simulink model "projeto_final_simulink"  (R2016a)
settings: Solver=VariableStepAuto  StartTime=0.0  StopTime=50  RelTol=1e-3
undefined symbols (not defined in the file): magnitude
settings Model: Creator=Luiz Renato  LastModifiedBy=Luiz Renato

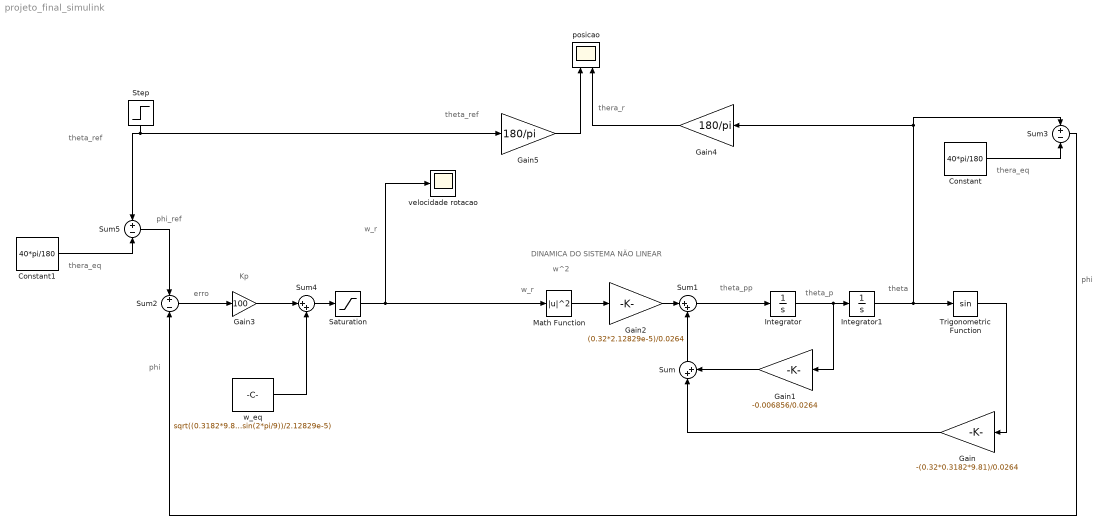
== system projeto_final_simulink ==
  note: DINAMICA DO SISTEMA NÃO LINEAR
  note: phi_ref
  note: phi
  note: erro
  note: theta_ref
  note: w^2
  note: w_r
  note: Kp
  note: theta_ref
  note: phi
  note: thera_eq
  note: thera_r
  note: w_r
  note: theta_pp
  note: theta_p
  note: theta
  note: thera_eq
  Constant : Constant  Value=40*pi/180
  Constant1 : Constant  Value=40*pi/180
  Gain : Gain  Gain=-(0.32*0.3182*9.81)/0.0264
  Gain1 : Gain  Gain=-0.006856/0.0264
  Gain2 : Gain  Gain=(0.32*2.12829e-5)/0.0264
  Gain3 : Gain  Gain=100
  Gain4 : Gain  Gain=180/pi
  Gain5 : Gain  Gain=180/pi
  Integrator : Integrator
  Integrator1 : Integrator
  Math Function : Math  Operator=magnitude^2  SaturateOnIntegerOverflow=on
  Saturation : Saturate  UpperLimit=375  LowerLimit=0
  Step : Step  Time=10  After=2*pi/9  SampleTime=0
  Sum : Sum  Inputs=|++
  Sum1 : Sum  Inputs=|++
  Sum2 : Sum  Inputs=+-
  Sum3 : Sum  Inputs=+-
  Sum4 : Sum  Inputs=|++
  Sum5 : Sum  Inputs=+-
  Trigonometric Function : Trigonometry
  posicao : Scope  NumInputPorts=2
  velocidade rotacao : Scope
  "w_eq " : Constant  Value=sqrt((0.3182*9.81*sin(2*pi/9))/2.12829e-5)
  wires:
  Integrator/1 -> Gain1/1, Integrator1/1
  Integrator1/1 -> Trigonometric Function/1, Sum3/1, Gain4/1
  Trigonometric Function/1 -> Gain/1
  Gain/1 -> Sum/1
  Gain1/1 -> Sum/2
  Sum1/1 -> Integrator/1
  Sum/1 -> Sum1/2
  Gain2/1 -> Sum1/1
  Constant/1 -> Sum3/2
  Sum3/1 -> Sum2/2
  Step/1 -> Gain5/1, Sum5/1
  Sum2/1 -> Gain3/1
  Gain3/1 -> Sum4/1
  "w_eq "/1 -> Sum4/2
  Sum4/1 -> Saturation/1
  Saturation/1 -> Math Function/1, velocidade rotacao/1
  Math Function/1 -> Gain2/1
  Gain4/1 -> posicao/2
  Gain5/1 -> posicao/1
  Constant1/1 -> Sum5/2
  Sum5/1 -> Sum2/1
